simulink model "Pitch_controller"  (R2020b)
settings: Solver=VariableStepAuto  StartTime=0.0  StopTime=10.0  RelTol=1e-3
values from neighbouring files (symbols this model uses):
  A_sp = [A_long_a_c(3:end,3) , A_long_a_c(3:end,4)]    [CAS_task6.m]    (also in SAS_task5.m)
  B_sp = [B_long_a_c(3:end)]    [CAS_task6.m]    (also in SAS_task5.m)
  C_sp = [C_long_a_c(3:end,3) , C_long_a_c(3:end,4)]    [CAS_task6.m]    (also in SAS_task5.m)
  K = place(A_sp,B_sp, poles_r)    [CAS_task6.m]    (also in SAS_task5.m)
  sys_sp = ss(A_sp,B_sp,C_sp,D_sp)    [CAS_task6.m]    (also in SAS_task5.m)
  tau_d = T_theta2_r    (= 0.162016784939)    [CAS_task6.m]    (also in SAS_task5.m)
  tau_i = T_theta2    [CAS_task6.m]    (also in SAS_task5.m)
settings Model: Creator=vladg  LastModifiedBy=vladg

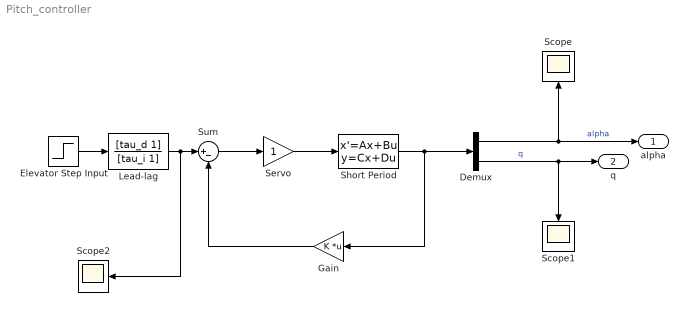
== system Pitch_controller ==
  Demux : Demux  Outputs=2
  Elevator Step Input : Step  SampleTime=0
  Gain : Gain  Gain=K  Multiplication=Matrix(K*u)
  Lead-lag : TransferFcn  Numerator=[tau_d 1]  Denominator=[tau_i 1]
  Scope : Scope
  Scope1 : Scope
  Scope2 : Scope
  Servo : Gain
  Short Period : StateSpace  A=A_sp  B=B_sp  C=C_sp  D=sys_sp.D  InitialCondition=0
  Sum : Sum  Inputs=|+-
  alpha : Outport
  q : Outport  Port=2
  wires:
  Short Period/1 -> Gain/1, Demux/1
  Demux/1 -> alpha/1, Scope/1  "alpha"
  Demux/2 -> Scope1/1, q/1  "q"
  Servo/1 -> Short Period/1
  Gain/1 -> Sum/2
  Sum/1 -> Servo/1
  Elevator Step Input/1 -> Lead-lag/1
  Lead-lag/1 -> Scope2/1, Sum/1
